simulink model "trenl"  (R2023a)
settings: Solver=VariableStepAuto  StartTime=0.0  StopTime=10.0  RelTol=1e-3
values from neighbouring files (symbols this model uses):
  n = zeros(1, N)    [main.m]    (also in matlab.mat = [2 6 1 2])
undefined symbols (not defined in the file or in its folder): m
settings Model: Creator=kelfi  LastModifiedBy=kelfi

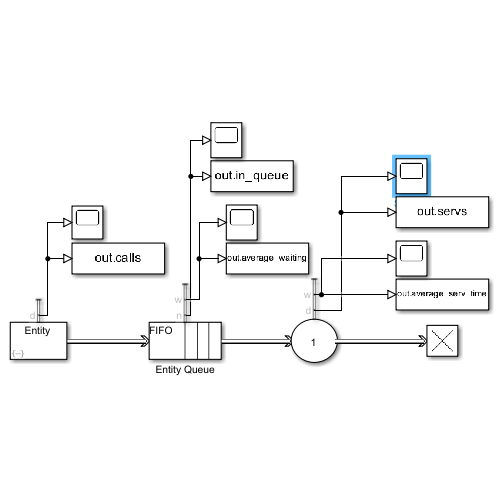
[thumbnail: Simulink's stored preview of the top-level diagram]
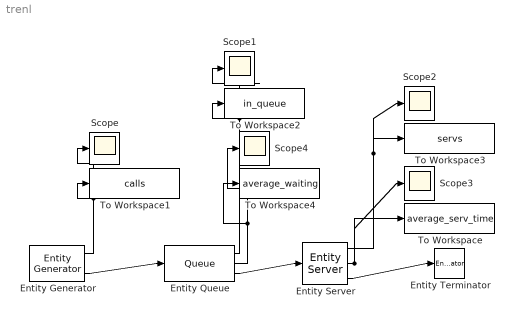
== system trenl ==
  Entity Generator : EntityGenerator  OutputPortMessageModes=n,m  TimeSource=MATLAB action  IntergenerationTimeAction=|  GenerateAction=|  AttributeName=patience  NumberEntitiesDeparted=on  EntityType=Structured  EntityTypeName=Entity
      | persistent rngInit;
      | if isempty(rngInit)
      |     seed = rand();
      |     rng(seed);
      |     rngInit = true;
      | end
      | 
      | mu = lambda;
      | dt = -mu * log(1 - rand());
      | persistent rngInit;
      | if isempty(rngInit)
      |     seed = 124124;
      |     rng(seed);
      |     rngInit = true;
      | end
      | 
      | entity.patience = randi([2, 5]);
      settings: OutputPortMap=o0,o3
  Entity Queue : Queue  InputPortMessageModes=m  OutputPortMessageModes=n,n,m  Capacity=inf  NumberEntitiesInBlock=on  AverageWait=on
      settings: OutputPortMap=o1,o2,o5
  Entity Server : EntityServer  InputPortMessageModes=m  OutputPortMessageModes=n,n,m  Capacity=1  ServiceTimeSource=MATLAB action  ServiceTimeAttributeName=sertime  ServiceTimeAction=|  NumberEntitiesDeparted=on  AverageWait=on
      | dt = rand(1,1);
      | persistent rngInit;
      | if isempty(rngInit)
      |     seed = rand();
      |     rng(seed);
      |     rngInit = true;
      | end
      | 
      | mu = t;
      | dt = -mu * log(1 - rand());
      settings: OutputPortMap=o0,o4,o9
  Entity Terminator : EntityTerminator  InputPortMessageModes=m
  Scope{,1..4} (5 alike) : Scope
  To Workspace : ToWorkspace  VariableName=average_serv_time  SampleTime=-1
      settings: MaxDataPoints=1
  To Workspace1 : ToWorkspace  VariableName=calls  SampleTime=-1
      settings: MaxDataPoints=1
  To Workspace2 : ToWorkspace  VariableName=in_queue  SampleTime=-1
      settings: MaxDataPoints=1
  To Workspace3 : ToWorkspace  VariableName=servs  SampleTime=-1
      settings: MaxDataPoints=1
  To Workspace4 : ToWorkspace  VariableName=average_waiting  SampleTime=-1
      settings: MaxDataPoints=1
  wires:
  Entity Generator/1 -> Scope/1, To Workspace1/1
  Entity Generator/2 -> Entity Queue/1
  Entity Server/3 -> Entity Terminator/1
  Entity Server/1 -> To Workspace3/1, Scope2/1
  Entity Queue/3 -> Entity Server/1
  Entity Server/2 -> Scope3/1, To Workspace/1
  Entity Queue/1 -> To Workspace2/1, Scope1/1
  Entity Queue/2 -> Scope4/1, To Workspace4/1
